simulink model "SIL_MIL"  (R2022b)
settings: Solver=FixedStepAuto  StartTime=0.0  StopTime=30  FixedStep=0.01  RelTol=1e-3
libraries: slpidlib x2, pil_lib x1
settings Model: Creator=ok  LastModifiedBy=ok
settings OptimizationCC: DefaultParameterBehavior=Inlined  EnhancedBackFolding=on  PassReuseOutputArgsAs=Individual arguments  ZeroExternalMemoryAtStartup=off  ZeroInternalMemoryAtStartup=off  OptimizeBlockOrder=speed  DifferentSizesBufferReuse=on  OptimizationCustomize=off  EfficientTunableParamExpr=on
settings DebuggingCC: ParameterTunabilityLossMsg=error
settings HardwareCC: ProdBitPerPointer=32  ProdBitPerSizeT=32  ProdBitPerPtrDiffT=32  ProdLargestAtomicFloat=None  ProdWordSize=32  ProdHWDeviceType=Atmel->AVR (32-bit)
settings SFSimCC: MATLABDynamicMemAlloc=off
settings RTWCC: Description=Embedded Coder  SystemTargetFile=ert.tlc  TemplateMakefile=ert_default_tmf
settings CodeAppCC: ForceParamTrailComments=on  IgnoreCustomStorageClasses=off  OperatorAnnotations=on  SimulinkDataObjDesc=on  SFDataObjDesc=on  InsertBlockDesc=on
settings ERTTargetCC: TargetLangStandard=C99 (ISO)  GenerateSampleERTMain=on  InlinedParameterPlacement=NonHierarchical  ERTCustomFileTemplate=example_file_process.tlc

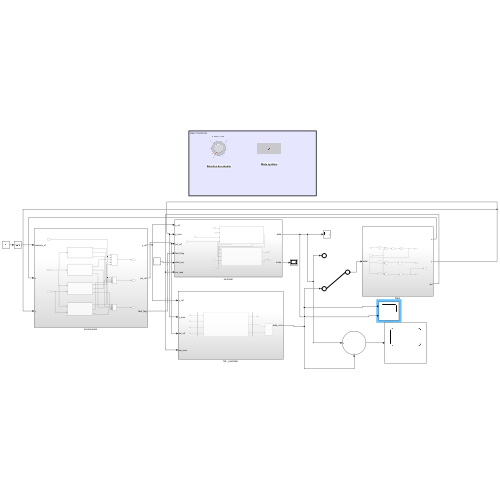
[thumbnail: Simulink's stored preview of the top-level diagram]
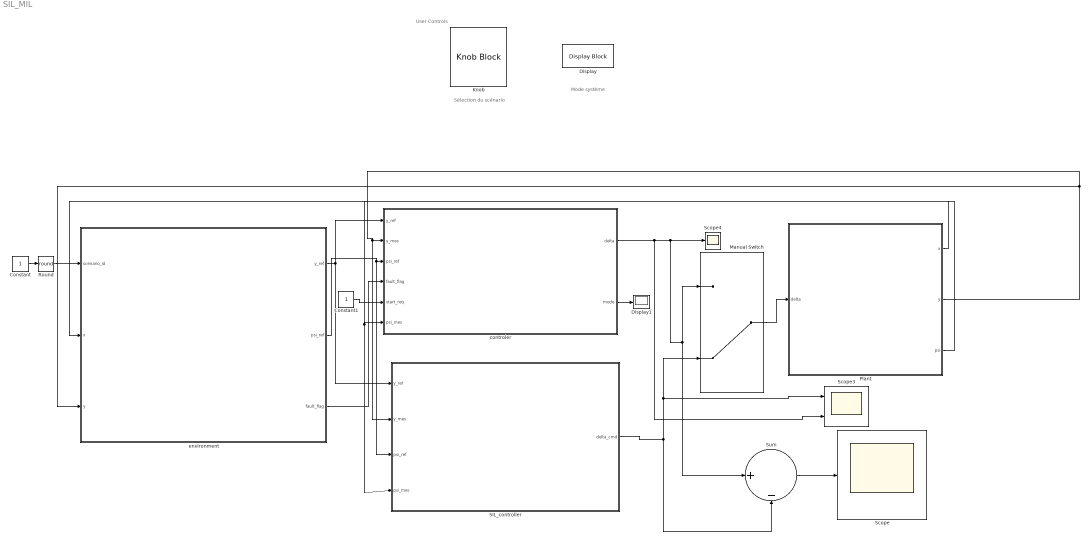
== system SIL_MIL ==
  note: Mode système
  note: Sélection du scénario
  note: User Controls
  Constant : Constant
  Constant1 : Constant
  Display : DisplayBlock  LabelPosition=Hide  Transparency=1
  Display1 : Display
  Knob : KnobBlock  ScaleMin=1  ScaleMax=4  TickInterval=1
  Manual Switch : ManualSwitch  CurrentSetting=0
  "Plant " : Subsystem
  Round : Rounding  Operator=round
  SIL_controller : Subsystem
  Scope : Scope
  Scope3 : Scope  NumInputPorts=2
  Scope4 : Scope
  Sum : Sum  Inputs=|+-
  controler : Subsystem
  "environment " : Subsystem
  wires:
  "environment "/3(fault_flag) -> controler/4(fault_flag)
  Manual Switch/1 -> "Plant "/1(delta)
  Sum/1 -> Scope/1
  controler/1(delta) -> Scope4/1, Sum/1, Manual Switch/1, Scope3/2
  Constant1/1 -> controler/5(start_req)
  Round/1 -> "environment "/1(scenario_id)
  "Plant "/2(y) -> SIL_controller/2(y_mes), controler/2(y_mes), "environment "/3(y)
  "Plant "/1(x) -> "environment "/2(x)
  "Plant "/3(psi) -> SIL_controller/4(psi_mes), controler/6(psi_mes)
  controler/2(mode) -> Display1/1
  Constant/1 -> Round/1
  "environment "/2(psi_ref) -> SIL_controller/3(psi_ref), controler/3(psi_ref)
  SIL_controller/1(delta_cmd) -> Sum/2, Manual Switch/2, Scope3/1
  "environment "/1(y_ref) -> controler/1(y_ref), SIL_controller/1(y_ref)

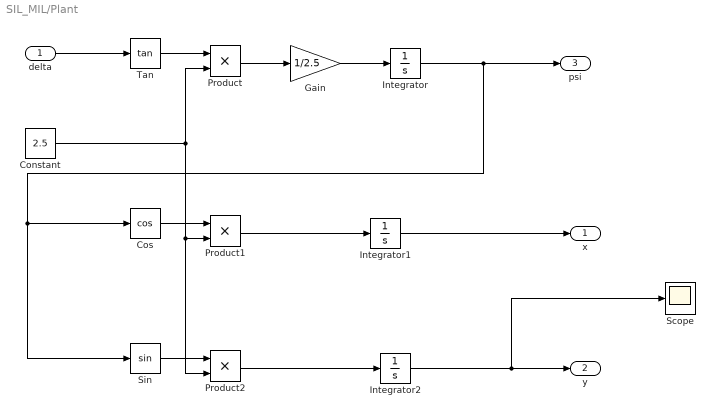
== system SIL_MIL/Plant  ==
  delta : Inport
  Constant : Constant  Value=2.5
  Cos : Trigonometry  Operator=cos
  Gain : Gain  Gain=1/2.5
  Integrator : Integrator
  Integrator1 : Integrator
  Integrator2 : Integrator
  Product : Product
  Product1 : Product
  Product2 : Product
  Scope : Scope
  Sin : Trigonometry
  Tan : Trigonometry  Operator=tan
  x : Outport
  y : Outport  Port=2
  psi : Outport  Port=3
  wires:
  delta/1 -> Tan/1
  Tan/1 -> Product/1
  Constant/1 -> Product/2, Product2/2, Product1/2
  Product/1 -> Gain/1
  Gain/1 -> Integrator/1
  Integrator/1 -> Sin/1, Cos/1, psi/1
  Cos/1 -> Product1/1
  Product1/1 -> Integrator1/1
  Integrator1/1 -> x/1
  Sin/1 -> Product2/1
  Product2/1 -> Integrator2/1
  Integrator2/1 -> Scope/1, y/1

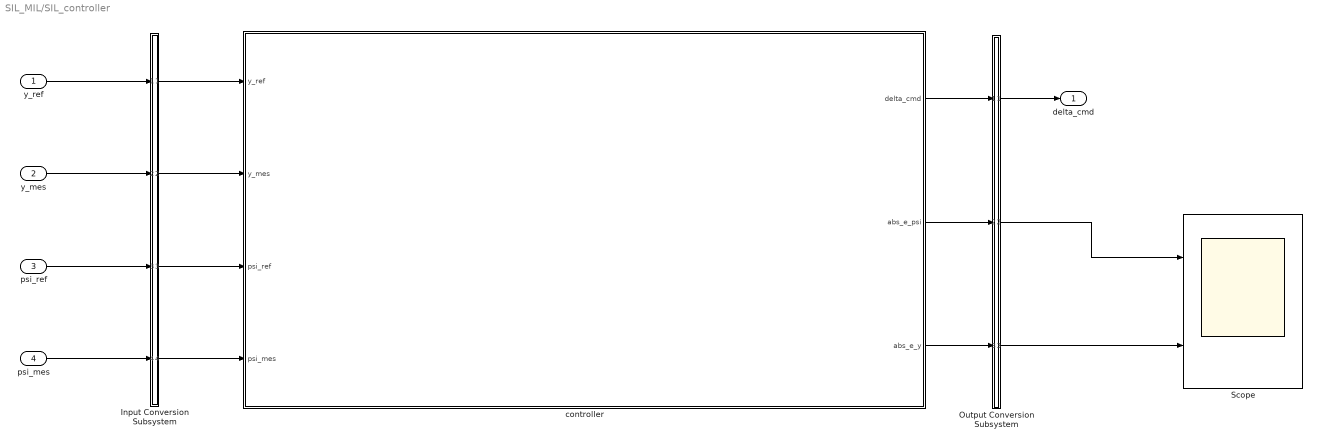
== system SIL_MIL/SIL_controller ==
  y_ref : Inport  OutDataTypeStr=double  PortDimensions=[1]  SampleTime=0
  y_mes : Inport  Port=2  OutDataTypeStr=double  PortDimensions=[1]  SampleTime=0
  psi_ref : Inport  Port=3  OutDataTypeStr=double  PortDimensions=[1]  SampleTime=0
  psi_mes : Inport  Port=4  OutDataTypeStr=double  PortDimensions=[1]  SampleTime=0
  Input Conversion Subsystem : Subsystem  Tag=__SLT_ICS__  Description=|
      | Signal spec.
      | and routing
      settings: AttributesFormatString=%<Description>
  Output Conversion Subsystem : Subsystem  Tag=__SLT_OCS__  Description=|
      | Signal spec.
      | and routing
      settings: AttributesFormatString=%<Description>
  Scope : Scope  NumInputPorts=2
  controller : Subsystem  Tag=__SL_testing_harness_stub_  DialogController=pil_create_dialog  LoadFcn=|
      | try
      |    if ~strcmp(rtw.pil.getPILVersion, '9.13 (R2022b)_15')
      |       set_param(gcb, 'DialogController', '');
      |       set_param(gcb, 'DialogControllerArgs', '');
      |    end
      | catch e
      |       set_param(gcb, 'DialogController', '');
      |       set_param(gcb, 'DialogControllerArgs', '');
      | end
      mask help: PIL:pil:XILBlockMaskDesc
      mask Display: disp('SIL');
  delta_cmd : Outport
  wires:
  Output Conversion Subsystem/1(Outport_1) -> delta_cmd/1
  Input Conversion Subsystem/4(Outport_4) -> controller/4(psi_mes)
  controller/3(abs_e_y) -> Output Conversion Subsystem/3(Inport_3)
  y_mes/1 -> Input Conversion Subsystem/2(Inport_2)
  y_ref/1 -> Input Conversion Subsystem/1(Inport_1)
  Input Conversion Subsystem/3(Outport_3) -> controller/3(psi_ref)
  Input Conversion Subsystem/2(Outport_2) -> controller/2(y_mes)
  controller/2(abs_e_psi) -> Output Conversion Subsystem/2(Inport_2)
  Input Conversion Subsystem/1(Outport_1) -> controller/1(y_ref)
  psi_mes/1 -> Input Conversion Subsystem/4(Inport_4)
  psi_ref/1 -> Input Conversion Subsystem/3(Inport_3)
  controller/1(delta_cmd) -> Output Conversion Subsystem/1(Inport_1)
  Output Conversion Subsystem/2(Outport_2) -> Scope/1
  Output Conversion Subsystem/3(Outport_3) -> Scope/2

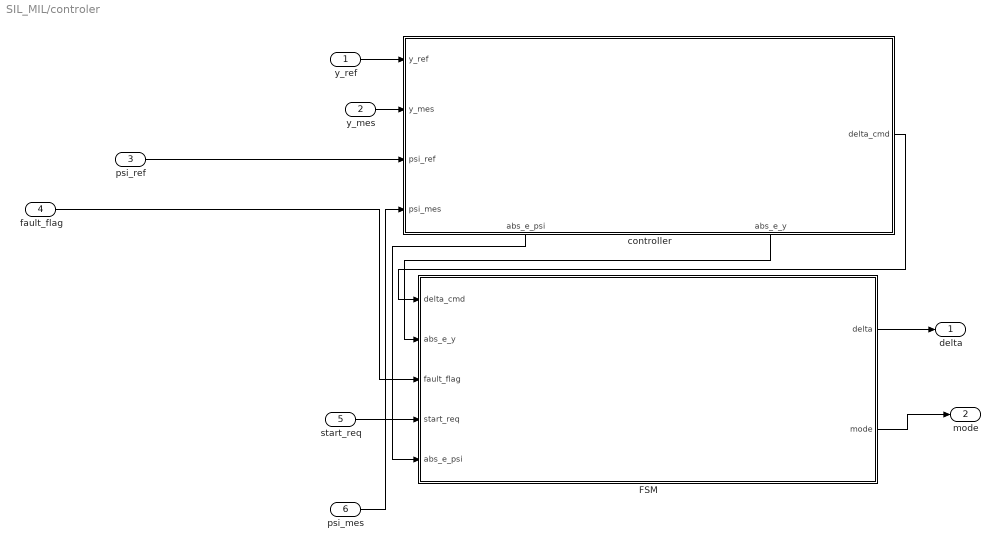
== system SIL_MIL/controler ==
  y_ref : Inport
  y_mes : Inport  Port=2
  psi_ref : Inport  Port=3
  fault_flag : Inport  Port=4
  start_req : Inport  Port=5
  psi_mes : Inport  Port=6
  FSM : Subsystem
  controller : Subsystem  TreatAsAtomicUnit=on
      settings: PortSchema="{\"entries\":[{\"content\":{\"sides\":[{\"content\":{\"connectorIds\":[\"In1\",\"In2\",\"In3\",\"In4\"]},\"type\":\"ConnectorPlacement.EquallySpacedRectSide\",\"uuid\":\"dce009df-b000-45c7-aa28-a3bb8a55b1fe\"},{\"content\":{\"connectorIds\":[\"Out1\"],\"side\":\"RIGHT\"},\"type\":\"ConnectorPlacement.EquallySpacedRectSide\",\"uuid\":\"27679ab1-5f7b-49ed-b0db-4270332b706f\"},{\"content\":{\"connectorIds\":[],\"side\":\"TOP\"},\"type\":\"ConnectorPlacement.EquallySpacedRectSide\",\"uuid\":\"474e0d2f-310b-4a94-af54-f468ed9e1b68\"},{\"content\":{\"connectorIds\":[\"Out2\",\"Out3\"],\"side\":\"BOTTOM\"},\"type\":\"ConnectorPlacement.EquallySpacedRectSide\",\"uuid\":\"e9194f37-6c87-4243-879e-6146eac92453\"}]},\"type\":\"ConnectorPlacement.EquallySpacedConnector\",\"uuid\":\"bf9faa3f-a673-4ccc-8b0a-d91001fa1506\"}],\"packageUris\":[\"http://schema.mathworks.com/mf0/Connector/R2020b\"],\"version\":\"1.0\"}"
  delta : Outport
  mode : Outport  Port=2
  wires:
  FSM/1(delta) -> delta/1
  controller/2(abs_e_psi) -> FSM/5(abs_e_psi)
  psi_ref/1 -> controller/3(psi_ref)
  fault_flag/1 -> FSM/3(fault_flag)
  controller/1(delta_cmd) -> FSM/1(delta_cmd)
  y_mes/1 -> controller/2(y_mes)
  controller/3(abs_e_y) -> FSM/2(abs_e_y)
  psi_mes/1 -> controller/4(psi_mes)
  start_req/1 -> FSM/4(start_req)
  FSM/2(mode) -> mode/1
  y_ref/1 -> controller/1(y_ref)

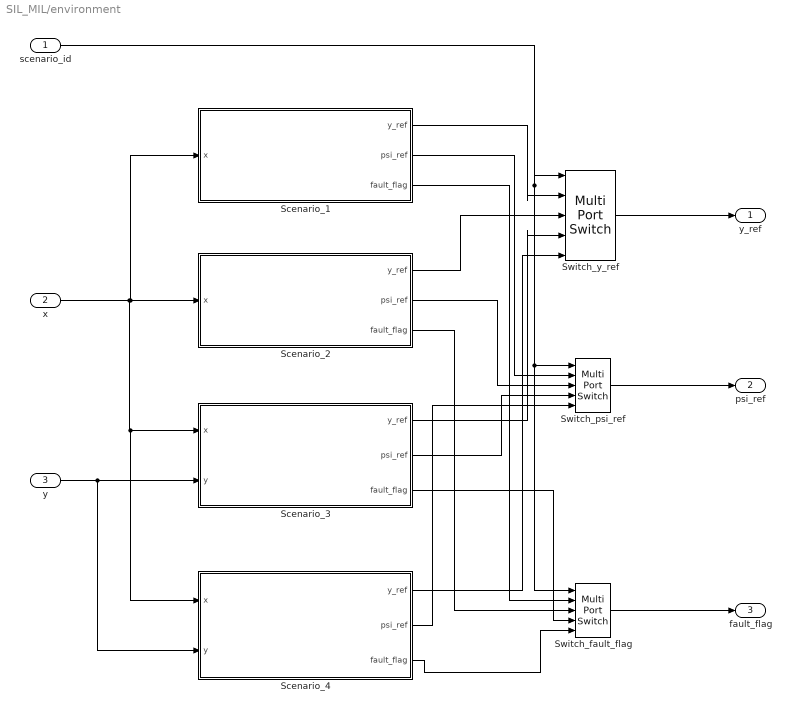
== system SIL_MIL/environment  ==
  scenario_id : Inport
  x : Inport  Port=2
  y : Inport  Port=3
  Scenario_1 : Subsystem
  Scenario_2 : Subsystem
  Scenario_3 : Subsystem
  Scenario_4 : Subsystem
  Switch_fault_flag : MultiPortSwitch  Inputs=4  SaturateOnIntegerOverflow=off  InputSameDT=off
  Switch_psi_ref : MultiPortSwitch  Inputs=4  SaturateOnIntegerOverflow=off  InputSameDT=off
  Switch_y_ref : MultiPortSwitch  Inputs=4  SaturateOnIntegerOverflow=off  InputSameDT=off
  y_ref : Outport
  psi_ref : Outport  Port=2
  fault_flag : Outport  Port=3
  wires:
  scenario_id/1 -> Switch_fault_flag/1, Switch_psi_ref/1, Switch_y_ref/1
  Scenario_1/1(y_ref) -> Switch_y_ref/2
  Scenario_2/1("y_ref ") -> Switch_y_ref/3
  Scenario_3/1("y_ref ") -> Switch_y_ref/4
  Scenario_4/1(y_ref) -> Switch_y_ref/5
  Scenario_1/2(psi_ref) -> Switch_psi_ref/2
  Scenario_2/2("psi_ref ") -> Switch_psi_ref/3
  Scenario_3/2("psi_ref ") -> Switch_psi_ref/4
  Scenario_4/2(psi_ref) -> Switch_psi_ref/5
  Scenario_1/3(fault_flag) -> Switch_fault_flag/2
  Scenario_2/3(fault_flag) -> Switch_fault_flag/3
  Scenario_3/3(fault_flag) -> Switch_fault_flag/4
  Scenario_4/3(fault_flag) -> Switch_fault_flag/5
  Switch_fault_flag/1 -> fault_flag/1
  Switch_psi_ref/1 -> psi_ref/1
  Switch_y_ref/1 -> y_ref/1
  x/1 -> Scenario_4/1(x), Scenario_3/1(x), Scenario_1/1(x), Scenario_2/1(x)
  y/1 -> Scenario_4/2(y), Scenario_3/2(y)

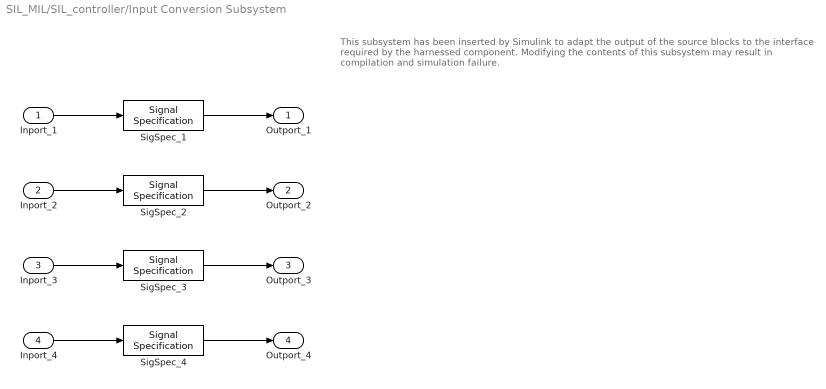
== system SIL_MIL/SIL_controller/Input Conversion Subsystem ==
  note: This subsystem has been inserted by Simulink to adapt the output of the source blocks to the interface required by the harnessed component.
      |  Modifying the contents of this subsystem may result in compilation and simulation failure.
  Inport_1 : Inport
  Inport_2 : Inport  Port=2
  Inport_3 : Inport  Port=3
  Inport_4 : Inport  Port=4
  SigSpec_{1..4} (4 alike) : SignalSpecification  OutDataTypeStr=double  Dimensions=[1]  SampleTime=[0, 0]
  Outport_1 : Outport
  Outport_2 : Outport  Port=2
  Outport_3 : Outport  Port=3
  Outport_4 : Outport  Port=4
  wires:
  SigSpec_1/1 -> Outport_1/1
  Inport_1/1 -> SigSpec_1/1
  SigSpec_2/1 -> Outport_2/1
  Inport_2/1 -> SigSpec_2/1
  SigSpec_3/1 -> Outport_3/1
  Inport_3/1 -> SigSpec_3/1
  SigSpec_4/1 -> Outport_4/1
  Inport_4/1 -> SigSpec_4/1

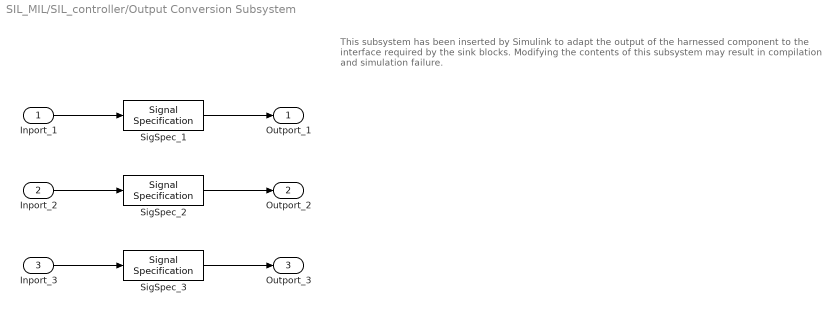
== system SIL_MIL/SIL_controller/Output Conversion Subsystem ==
  note: This subsystem has been inserted by Simulink to adapt the output of the harnessed component to the interface required by the sink blocks.
      |  Modifying the contents of this subsystem may result in compilation and simulation failure.
  Inport_1 : Inport
  Inport_2 : Inport  Port=2
  Inport_3 : Inport  Port=3
  SigSpec_1 : SignalSpecification  OutDataTypeStr=double  Dimensions=[1]  SampleTime=0.01
  SigSpec_2 : SignalSpecification  OutDataTypeStr=double  Dimensions=[1]
  SigSpec_3 : SignalSpecification  OutDataTypeStr=double  Dimensions=[1]
  Outport_1 : Outport
  Outport_2 : Outport  Port=2
  Outport_3 : Outport  Port=3
  wires:
  Inport_1/1 -> SigSpec_1/1
  SigSpec_1/1 -> Outport_1/1
  Inport_2/1 -> SigSpec_2/1
  SigSpec_2/1 -> Outport_2/1
  Inport_3/1 -> SigSpec_3/1
  SigSpec_3/1 -> Outport_3/1

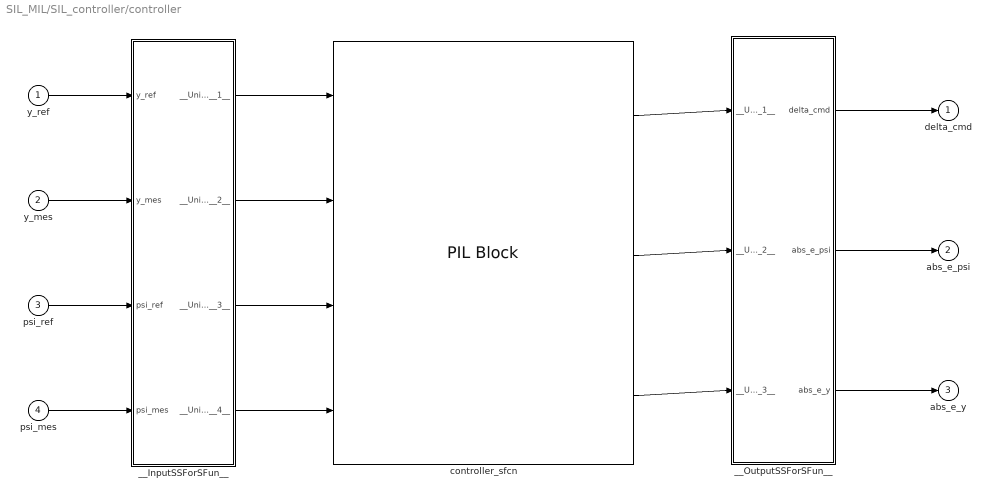
== system SIL_MIL/SIL_controller/controller ==
  y_ref : Inport
  y_mes : Inport  Port=2
  psi_ref : Inport  Port=3
  psi_mes : Inport  Port=4
  __InputSSForSFun__ : Subsystem
  __OutputSSForSFun__ : Subsystem
  controller_sfcn : pil_lib/PIL Block  SimulationMode=SIL  IsTopModelPIL=off  CodeDir=controller_ert_rtw  AnchorDir=C:\Users\ok\Documents\retest  ConfigName=Software-in-the-Loop (SIL)  XrelIsTopModelCode=on  XrelIsReusable=off  XrelDWorkNames={}  XrelDWorkTypes={}  XrelModelArgVals={}  XrelOrderedParamNames={}
  delta_cmd : Outport
  abs_e_psi : Outport  Port=2
  abs_e_y : Outport  Port=3
  wires:
  __OutputSSForSFun__/3(abs_e_y) -> abs_e_y/1
  __OutputSSForSFun__/2(abs_e_psi) -> abs_e_psi/1
  __OutputSSForSFun__/1(delta_cmd) -> delta_cmd/1
  controller_sfcn/3 -> __OutputSSForSFun__/3(__UniqueInportName__3__)
  controller_sfcn/2 -> __OutputSSForSFun__/2(__UniqueInportName__2__)
  controller_sfcn/1 -> __OutputSSForSFun__/1(__UniqueInportName__1__)
  __InputSSForSFun__/4(__UniqueOutportName__4__) -> controller_sfcn/4
  __InputSSForSFun__/3(__UniqueOutportName__3__) -> controller_sfcn/3
  __InputSSForSFun__/2(__UniqueOutportName__2__) -> controller_sfcn/2
  __InputSSForSFun__/1(__UniqueOutportName__1__) -> controller_sfcn/1
  psi_mes/1 -> __InputSSForSFun__/4(psi_mes)
  psi_ref/1 -> __InputSSForSFun__/3(psi_ref)
  y_mes/1 -> __InputSSForSFun__/2(y_mes)
  y_ref/1 -> __InputSSForSFun__/1(y_ref)

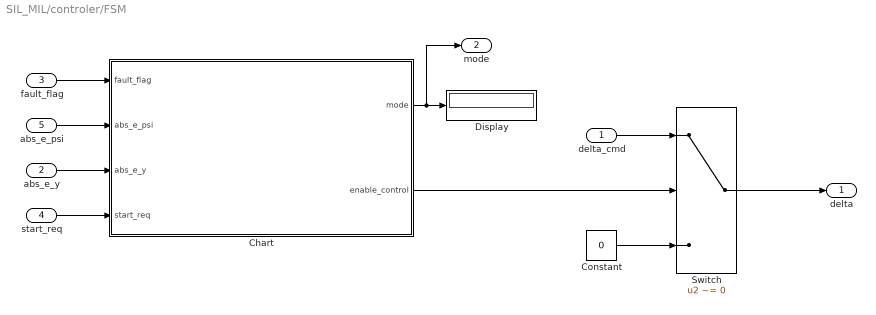
== system SIL_MIL/controler/FSM ==
  delta_cmd : Inport
  abs_e_y : Inport  Port=2
  fault_flag : Inport  Port=3
  start_req : Inport  Port=4
  abs_e_psi : Inport  Port=5
  Chart : Stateflow chart  TreatAsAtomicUnit=on
  Constant : Constant  Value=0
  Display : Display
  Switch : Switch  Criteria=u2 ~= 0  SaturateOnIntegerOverflow=off  InputSameDT=off
  delta : Outport
  mode : Outport  Port=2
  wires:
  Chart/1(mode) -> mode/1, Display/1
  delta_cmd/1 -> Switch/1
  Switch/1 -> delta/1
  Chart/2(enable_control) -> Switch/2
  Constant/1 -> Switch/3
  abs_e_y/1 -> Chart/3(abs_e_y)
  fault_flag/1 -> Chart/1(fault_flag)
  abs_e_psi/1 -> Chart/2(abs_e_psi)
  start_req/1 -> Chart/4(start_req)

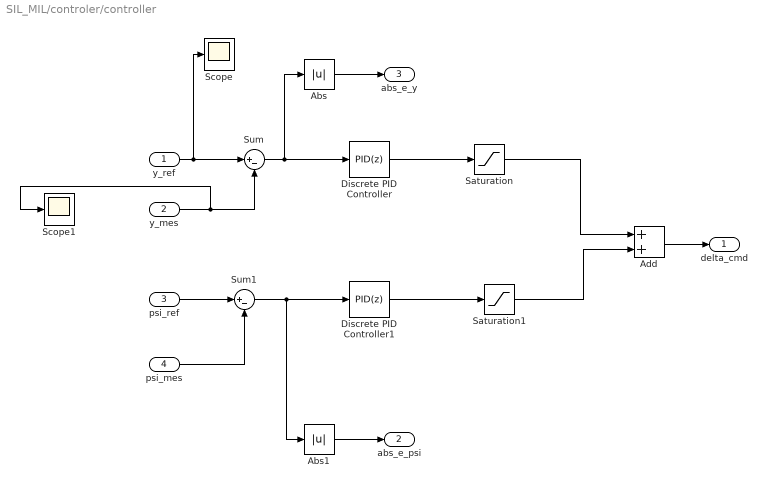
== system SIL_MIL/controler/controller ==
  y_ref : Inport
  y_mes : Inport  Port=2
  psi_ref : Inport  Port=3
  psi_mes : Inport  Port=4
  Abs : Abs  SaturateOnIntegerOverflow=off
  Abs1 : Abs  SaturateOnIntegerOverflow=off
  Add : Sum
  Discrete PID Controller : slpidlib/PID Controller  Controller=PID  Form=Parallel  TimeDomain=Discrete-time  UseExternalTs=off  SampleTime=-1  IntegratorMethod=Forward Euler  FilterMethod=Forward Euler  ControllerParametersSource=internal  P=1  I=1  UseKiTs=off  D=0  N=100  UseFilter=on  TunerSelectOption=Transfer Function Based (PID Tuner App)  InitialConditionSource=internal  InitialConditionForIntegrator=0  InitialConditionForFilter=0  DifferentiatorICPrevScaledInput=0  ExternalReset=none  TrackingMode=off  Kt=1  LimitOutput=off  SatLimitsSource=internal  UpperSaturationLimit=inf  LowerSaturationLimit=-inf  LinearizeAsGain=off  AntiWindupMode=none  Kb=1  LimitIntegrator=off  UpperIntegratorSaturationLimit=inf  LowerIntegratorSaturationLimit=-inf  POutMin=[]  POutMax=[]  IOutMin=[]  IOutMax=[]  DOutMin=[]  DOutMax=[]  NOutMin=[]  NOutMax=[]  SumOutMin=[]  SumOutMax=[]  SaturationOutMin=[]  SaturationOutMax=[]  PParamMin=[]  PParamMax=[]  IParamMin=[]  IParamMax=[]  DParamMin=[]  DParamMax=[]  NParamMin=[]  NParamMax=[]  KbParamMin=[]  KbParamMax=[]  KtParamMin=[]  KtParamMax=[]  KbOutMin=[]  KbOutMax=[]  KtOutMin=[]  KtOutMax=[]  IntegratorOutMin=[]  IntegratorOutMax=[]  FilterOutMin=[]  FilterOutMax=[]  SumI1OutMin=[]  SumI1OutMax=[]  SumI2OutMin=[]  SumI2OutMax=[]  SumI3OutMin=[]  SumI3OutMax=[]  SumI4OutMin=[]  SumI4OutMax=[]  SumDOutMin=[]  SumDOutMax=[]  DifferentiatorOutMin=[]  DifferentiatorOutMax=[]  FilterDiffOutCoefMin=[]  FilterDiffOutCoefMax=[]  ReciprocalOutMin=[]  ReciprocalOutMax=[]  SumDenOutMin=[]  SumDenOutMax=[]  SumNumOutMin=[]  SumNumOutMax=[]  DivideOutMin=[]  DivideOutMax=[]  UdiffTsProdOutMin=[]  UdiffTsProdOutMax=[]  NTsProdOutMin=[]  NTsProdOutMax=[]  UintegralTsProdOutMin=[]  UintegralTsProdOutMax=[]  UngainTsProdOutMin=[]  UngainTsProdOutMax=[]  ClampingZeroOutDataTypeStr=Inherit: Inherit via back propagation  ClampingZeroOutMin=[]  ClampingZeroOutMax=[]  FilterDenConstantOutDataTypeStr=Inherit: Inherit via back propagation  FilterDenConstantOutMin=[]  FilterDenConstantOutMax=[]  PCopyOutDataTypeStr=Inherit: Inherit via back propagation  PCopyOutMin=[]  PCopyOutMax=[]  NCopyOutDataTypeStr=Inherit: Inherit via back propagation  NCopyOutMin=[]  NCopyOutMax=[]  IntegratorContinuousStateAttributes=''  IntegratorStateMustResolveToSignalObject=off  IntegratorRTWStateStorageClass=Auto  FilterContinuousStateAttributes=''  FilterStateMustResolveToSignalObject=off  FilterRTWStateStorageClass=Auto  ParallelPVariant=InternalParameters  IdealPVariant=Disabled  IVariant=InternalParameters  DVariant=InternalParameters  IntegratorVariant=Discrete  SatVariant=Disabled  AWVariant=Passthrough  PCopyVariant=Disabled  TRVariant=Disabled  FdbkBlocksVariant=Forward  IdealPFdbkVariant=Disabled  SatFdbkVariant=Disabled  DerivativeFilterVariant=ForwardEulerFilter  NVariant=InternalParameters  NCopyVariant=Disabled  FilterICVariant=InternalICsFilter  IntegratorICVariant=InternalICs  ExternalResetVariant=Disabled  TRSumVariant=Passthrough  SumFdbkVariant=Disabled  SumVariant=Sum_PID  TsampFilterVariant=InternalTs  TsampNgainVariant=Passthrough  TsampIntegralVariant=Passthrough  ExternalSaturationOutDataTypeStr=Inherit: Same as second input
      settings: LibrarySourceBlock=simulink/Discrete/Discrete PID Controller
  Discrete PID Controller1 : slpidlib/PID Controller  Controller=PID  Form=Parallel  TimeDomain=Discrete-time  UseExternalTs=off  SampleTime=-1  IntegratorMethod=Forward Euler  FilterMethod=Forward Euler  ControllerParametersSource=internal  P=1  I=1  UseKiTs=off  D=0  N=100  UseFilter=on  TunerSelectOption=Transfer Function Based (PID Tuner App)  InitialConditionSource=internal  InitialConditionForIntegrator=0  InitialConditionForFilter=0  DifferentiatorICPrevScaledInput=0  ExternalReset=none  TrackingMode=off  Kt=1  LimitOutput=off  SatLimitsSource=internal  UpperSaturationLimit=inf  LowerSaturationLimit=-inf  LinearizeAsGain=off  AntiWindupMode=none  Kb=1  LimitIntegrator=off  UpperIntegratorSaturationLimit=inf  LowerIntegratorSaturationLimit=-inf  POutMin=[]  POutMax=[]  IOutMin=[]  IOutMax=[]  DOutMin=[]  DOutMax=[]  NOutMin=[]  NOutMax=[]  SumOutMin=[]  SumOutMax=[]  SaturationOutMin=[]  SaturationOutMax=[]  PParamMin=[]  PParamMax=[]  IParamMin=[]  IParamMax=[]  DParamMin=[]  DParamMax=[]  NParamMin=[]  NParamMax=[]  KbParamMin=[]  KbParamMax=[]  KtParamMin=[]  KtParamMax=[]  KbOutMin=[]  KbOutMax=[]  KtOutMin=[]  KtOutMax=[]  IntegratorOutMin=[]  IntegratorOutMax=[]  FilterOutMin=[]  FilterOutMax=[]  SumI1OutMin=[]  SumI1OutMax=[]  SumI2OutMin=[]  SumI2OutMax=[]  SumI3OutMin=[]  SumI3OutMax=[]  SumI4OutMin=[]  SumI4OutMax=[]  SumDOutMin=[]  SumDOutMax=[]  DifferentiatorOutMin=[]  DifferentiatorOutMax=[]  FilterDiffOutCoefMin=[]  FilterDiffOutCoefMax=[]  ReciprocalOutMin=[]  ReciprocalOutMax=[]  SumDenOutMin=[]  SumDenOutMax=[]  SumNumOutMin=[]  SumNumOutMax=[]  DivideOutMin=[]  DivideOutMax=[]  UdiffTsProdOutMin=[]  UdiffTsProdOutMax=[]  NTsProdOutMin=[]  NTsProdOutMax=[]  UintegralTsProdOutMin=[]  UintegralTsProdOutMax=[]  UngainTsProdOutMin=[]  UngainTsProdOutMax=[]  ClampingZeroOutDataTypeStr=Inherit: Inherit via back propagation  ClampingZeroOutMin=[]  ClampingZeroOutMax=[]  FilterDenConstantOutDataTypeStr=Inherit: Inherit via back propagation  FilterDenConstantOutMin=[]  FilterDenConstantOutMax=[]  PCopyOutDataTypeStr=Inherit: Inherit via back propagation  PCopyOutMin=[]  PCopyOutMax=[]  NCopyOutDataTypeStr=Inherit: Inherit via back propagation  NCopyOutMin=[]  NCopyOutMax=[]  IntegratorContinuousStateAttributes=''  IntegratorStateMustResolveToSignalObject=off  IntegratorRTWStateStorageClass=Auto  FilterContinuousStateAttributes=''  FilterStateMustResolveToSignalObject=off  FilterRTWStateStorageClass=Auto  ParallelPVariant=InternalParameters  IdealPVariant=Disabled  IVariant=InternalParameters  DVariant=InternalParameters  IntegratorVariant=Discrete  SatVariant=Disabled  AWVariant=Passthrough  PCopyVariant=Disabled  TRVariant=Disabled  FdbkBlocksVariant=Forward  IdealPFdbkVariant=Disabled  SatFdbkVariant=Disabled  DerivativeFilterVariant=ForwardEulerFilter  NVariant=InternalParameters  NCopyVariant=Disabled  FilterICVariant=InternalICsFilter  IntegratorICVariant=InternalICs  ExternalResetVariant=Disabled  TRSumVariant=Passthrough  SumFdbkVariant=Disabled  SumVariant=Sum_PID  TsampFilterVariant=InternalTs  TsampNgainVariant=Passthrough  TsampIntegralVariant=Passthrough  ExternalSaturationOutDataTypeStr=Inherit: Same as second input
      settings: LibrarySourceBlock=simulink/Discrete/Discrete PID Controller
  Saturation : Saturate
  Saturation1 : Saturate
  Scope : Scope
  Scope1 : Scope
  Sum : Sum  Inputs=|+-
  Sum1 : Sum  Inputs=|+-
  delta_cmd : Outport
  abs_e_psi : Outport  Port=2
  abs_e_y : Outport  Port=3
  wires:
  y_ref/1 -> Scope/1, Sum/1
  y_mes/1 -> Scope1/1, Sum/2
  Sum/1 -> Discrete PID Controller/1, Abs/1
  psi_ref/1 -> Sum1/1
  psi_mes/1 -> Sum1/2
  Discrete PID Controller/1 -> Saturation/1
  Sum1/1 -> Discrete PID Controller1/1, Abs1/1
  Discrete PID Controller1/1 -> Saturation1/1
  Add/1 -> delta_cmd/1
  Saturation/1 -> Add/1
  Saturation1/1 -> Add/2
  Abs/1 -> abs_e_y/1
  Abs1/1 -> abs_e_psi/1

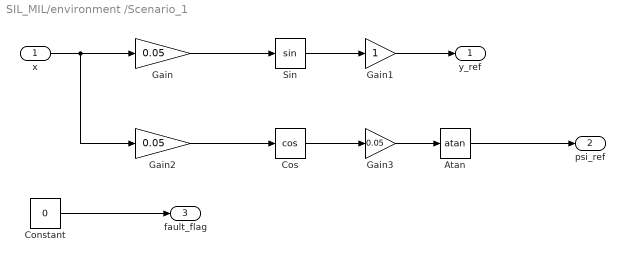
== system SIL_MIL/environment /Scenario_1 ==
  x : Inport
  Atan : Trigonometry  Operator=atan
  Constant : Constant  Value=0
  Cos : Trigonometry  Operator=cos
  Gain : Gain  Gain=0.05
  Gain1 : Gain
  Gain2 : Gain  Gain=0.05
  Gain3 : Gain  Gain=0.05
  Sin : Trigonometry
  y_ref : Outport
  psi_ref : Outport  Port=2
  fault_flag : Outport  Port=3
  wires:
  x/1 -> Gain2/1, Gain/1
  Gain/1 -> Sin/1
  Sin/1 -> Gain1/1
  Gain1/1 -> y_ref/1
  Cos/1 -> Gain3/1
  Gain2/1 -> Cos/1
  Gain3/1 -> Atan/1
  Atan/1 -> psi_ref/1
  Constant/1 -> fault_flag/1

== system SIL_MIL/environment /Scenario_2 ==
  x : Inport
  MATLAB Function : MATLAB Function  TreatAsAtomicUnit=on
  "y_ref " : Outport
  "psi_ref " : Outport  Port=2
  fault_flag : Outport  Port=3
  wires:
  MATLAB Function/1(y_ref) -> "y_ref "/1
  MATLAB Function/2(psi_ref) -> "psi_ref "/1
  MATLAB Function/3(fault_flag) -> fault_flag/1
  x/1 -> MATLAB Function/1(x)

== system SIL_MIL/environment /Scenario_3 ==
  x : Inport
  y : Inport  Port=2
  MATLAB Function : MATLAB Function  TreatAsAtomicUnit=on
  "y_ref " : Outport
  "psi_ref " : Outport  Port=2
  fault_flag : Outport  Port=3
  wires:
  MATLAB Function/1(y_ref) -> "y_ref "/1
  MATLAB Function/3(fault_flag) -> fault_flag/1
  y/1 -> MATLAB Function/2(y)
  MATLAB Function/2(psi_ref) -> "psi_ref "/1
  x/1 -> MATLAB Function/1(x)

== system SIL_MIL/environment /Scenario_4 ==
  x : Inport
  y : Inport  Port=2
  MATLAB Function : MATLAB Function  TreatAsAtomicUnit=on
  y_ref : Outport
  psi_ref : Outport  Port=2
  fault_flag : Outport  Port=3
  wires:
  x/1 -> MATLAB Function/1(x)
  MATLAB Function/1(y_ref) -> y_ref/1
  MATLAB Function/2(psi_ref) -> psi_ref/1
  MATLAB Function/3(fault_flag) -> fault_flag/1
  y/1 -> MATLAB Function/2(y)

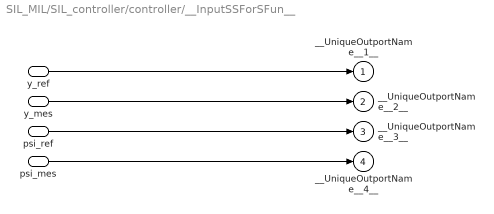
== system SIL_MIL/SIL_controller/controller/__InputSSForSFun__ ==
  y_ref : Inport
  y_mes : Inport  Port=2
  psi_ref : Inport  Port=3
  psi_mes : Inport  Port=4
  __UniqueOutportName__1__ : Outport
  __UniqueOutportName__2__ : Outport  Port=2
  __UniqueOutportName__3__ : Outport  Port=3
  __UniqueOutportName__4__ : Outport  Port=4
  wires:
  psi_mes/1 -> __UniqueOutportName__4__/1
  psi_ref/1 -> __UniqueOutportName__3__/1
  y_mes/1 -> __UniqueOutportName__2__/1
  y_ref/1 -> __UniqueOutportName__1__/1

== system SIL_MIL/SIL_controller/controller/__OutputSSForSFun__ ==
  __UniqueInportName__1__ : Inport
  __UniqueInportName__2__ : Inport  Port=2
  __UniqueInportName__3__ : Inport  Port=3
  delta_cmd : Outport
  abs_e_psi : Outport  Port=2
  abs_e_y : Outport  Port=3
  wires:
  __UniqueInportName__3__/1 -> abs_e_y/1
  __UniqueInportName__2__/1 -> abs_e_psi/1
  __UniqueInportName__1__/1 -> delta_cmd/1

== matlab function SIL_MIL/environment /Scenario_3/MATLAB Function ==
  data: x input; y_ref output; y input; psi_ref output; fault_flag output
function [y_ref, psi_ref, fault_flag] = scenario3_onecurve(x, y)
%#codegen

% Paramètres de la route
A = 2.0;      % amplitude de la courbe
xc = 25.0;    % centre de la courbe
sigma = 6.0;  % largeur de la courbe

% Référence latérale : une seule bosse douce
dx = x - xc;
y_ref = A * exp(-(dx*dx)/(2*sigma*sigma));

% Dérivée par rapport à x
dy_dx = y_ref * ( -dx / (sigma*sigma) );

% Orientation de référence
psi_ref = atan(dy_dx);

% Pas de défaut dans ce scénario
fault_flag = 0;

== matlab function SIL_MIL/environment /Scenario_2/MATLAB Function ==
  data: x input; y_ref output; psi_ref output; fault_flag output
function [y_ref, psi_ref, fault_flag] = environment_fun(x)
%#codegen

% Route sinueuse simple et cohérente
A = 2;       % amplitude
B = 0.1;     % fréquence spatiale

y_ref = A*sin(B*x);

% pente de la route
dy_dx = A*B*cos(B*x);

% orientation de la route
psi_ref = atan(dy_dx);

% défaut
fault_flag = 0;

end

== stateflow chart SIL_MIL/controler/FSM/Chart ==
  state Init
    en:
    enable_control = 0;
    mode = 0;
  state Nominal
    en:
    enable_control = 1;
    mode = 2;
  state Standby
    en:
    enable_control = 0;
    mode = 1;
  state Emergency
    en:
    enable_control = 0;
    mode = 3;
  (default) -> Init
  Standby -> Nominal : [start_req == 1 && fault_flag == 0]
  Init -> Standby : after(0.5,sec)
  Emergency -> Standby : [start_req == 0 && fault_flag == 0]
  Nominal -> Emergency : [fault_flag == 1 || abs_e_y > 1.5 || abs_e_psi > 0.5]
  data: mode output; enable_control output; fault_flag input; abs_e_psi input; abs_e_y input; start_req input

== matlab function SIL_MIL/environment /Scenario_4/MATLAB Function ==
  data: x input; y_ref output; psi_ref output; fault_flag output; y input
function [y_ref, psi_ref, fault_flag] = scenario4_simple(x, y)
%#codegen
% Scenario 4 : sinusoide puis virage

A = 2;        % amplitude sinusoide
B = 0.08;     % frequence
x_turn = 60;  % point ou on tourne

if x < x_turn
    
    % ===== PARTIE 1 : SINUSOIDE =====
    y_ref = A * sin(B*x);
    dy_dx = A * B * cos(B*x);

else
    
    % ===== PARTIE 2 : VIRAGE CLAIR =====
    R = 20;   % rayon du virage
    
    dx = x - x_turn;
    
    % courbe type parabole (simple et stable)
    y_ref = A * sin(B*x_turn) + (dx^2)/(2*R);
    
    dy_dx = dx / R;

end

% orientation
psi_ref = atan(dy_dx);

% pas de defaut
fault_flag = 0;
